simulink model "Masa_Resorte_Amortiguador"  (R2017a)
settings: Solver=VariableStepAuto  StartTime=0.0  StopTime=120  RelTol=1e-3
InitFcn:
  | m=7
  | b=0.5
  | k=1.2
  | F=0
StartFcn:
  | m=2
  | b=0.5
  | k=1
settings Model: Creator=LuisFernando  LastModifiedBy=LuisFernando

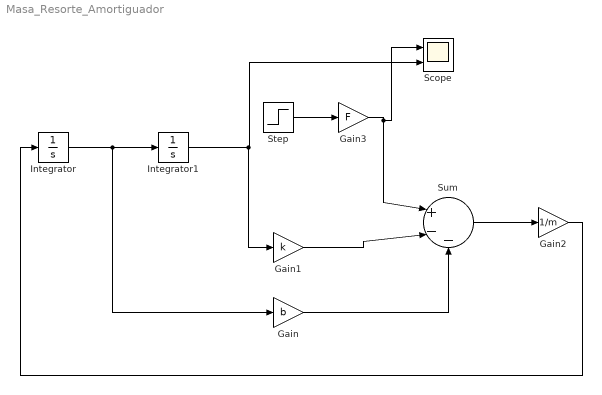
== system Masa_Resorte_Amortiguador ==
  Gain : Gain  Gain=b
  Gain1 : Gain  Gain=k
  Gain2 : Gain  Gain=1/m
  Gain3 : Gain  Gain=F
  Integrator : Integrator  InitialCondition=1
  Integrator1 : Integrator  InitialCondition=2
  Scope : Scope  NumInputPorts=2
  Step : Step  SampleTime=0
  Sum : Sum  Inputs=|+--
  wires:
  Integrator/1 -> Integrator1/1, Gain/1
  Step/1 -> Gain3/1
  Gain3/1 -> Scope/1, Sum/1
  Gain1/1 -> Sum/2
  Gain/1 -> Sum/3
  Sum/1 -> Gain2/1
  Gain2/1 -> Integrator/1
  Integrator1/1 -> Gain1/1, Scope/2
